simulink model "cameraUseModel"  (R2016a)
settings: Solver=ode15s  StartTime=0.0  StopTime=0.1  RelTol=1e-3
settings Model: Creator=mnorrito  LastModifiedBy=mnorrito

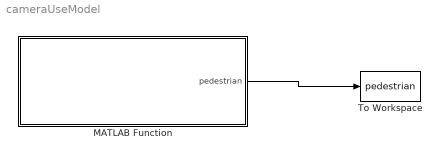
== system cameraUseModel ==
  MATLAB Function : MATLAB Function  TreatAsAtomicUnit=on
  To Workspace : ToWorkspace  VariableName=pedestrian  SaveFormat=Timeseries  SampleTime=-1
  wires:
  MATLAB Function/1(pedestrian) -> To Workspace/1

== matlab function cameraUseModel/MATLAB Function ==
  data: pedestrian output
function pedestrian  = cameraUseModel()
coder.extrinsic('evalin')
coder.extrinsic('imageUse')

img = evalin('base','cameraImage');
cn = 640;
ln = 480;
pedestrian = 0;

pedestrian = imageUse(ln, cn, img);

end
